simulink model "ir_info_sim"  (R2016a)
settings: Solver=FixedStepAuto  StartTime=0.0  StopTime=20  FixedStep=0.01  RelTol=1e-3
settings Model: Creator=maximilian  LastModifiedBy=maximilian

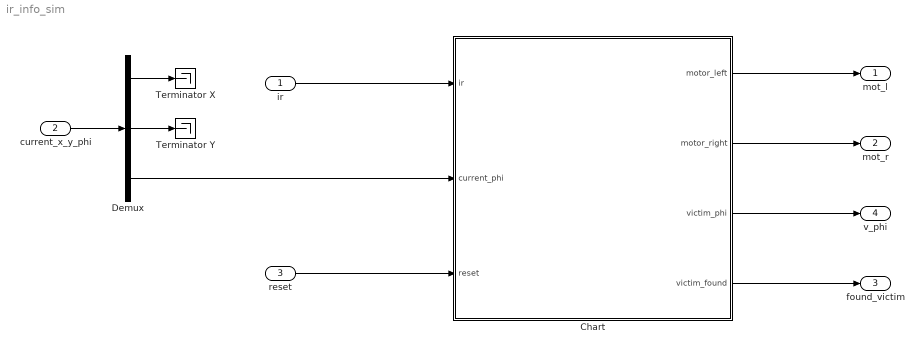
== system ir_info_sim ==
  ir : Inport  PortDimensions=[6]
  current_x_y_phi : Inport  Port=2  PortDimensions=[3]
  reset : Inport  Port=3
  Chart : Stateflow chart  TreatAsAtomicUnit=on
  Demux : Demux  Outputs=3
  Terminator X : Terminator
  Terminator Y : Terminator
  mot_l : Outport
  mot_r : Outport  Port=2
  found_victim : Outport  Port=3
  v_phi : Outport  Port=4
  wires:
  Chart/1(motor_left) -> mot_l/1
  Chart/2(motor_right) -> mot_r/1
  Chart/3(victim_phi) -> v_phi/1
  Chart/4(victim_found) -> found_victim/1
  ir/1 -> Chart/1(ir)
  reset/1 -> Chart/3(reset)
  current_x_y_phi/1 -> Demux/1
  Demux/3 -> Chart/2(current_phi)
  Demux/1 -> Terminator X/1
  Demux/2 -> Terminator Y/1

== stateflow chart ir_info_sim/Chart ==
  state Start
    entry:
    % Precondition: At least one sensor
    % deos not detect an IR signal.
    victim_found = 0;
    sonsor = -1
    for i = 1:6
    if ir(i) == 0
    sensor = i;
    end
    end
    motor_left = -1;
    motor_right = 1;
  state Bound1
    entry:
    bound1 = current_phi;
  state End
    entry:
    victim_phi = mod(current_phi - bound1, 2 * pi);
    victim_found = 1;
  (default) -> Start
  Start -> Start [order 2] : [reset == 1]
  End -> Start : [reset == 1]
  Bound1 -> Start [order 2] : [reset == 1]
  Start -> Bound1 [order 1] : [ir(sensor) == 1]
  Bound1 -> End [order 1] : [ir(sensor) == 0]
  data: motor_left output; ir input; current_phi input; motor_right output; victim_phi output; victim_found output; sonsor local; bound1 local; i local; sensor local; reset input
